simulink model "ES101A_DiagcMgrProxyX"  (R2013b)
settings: Solver=ode45  StartTime=0.0  StopTime=10.0  RelTol=1e-3
values from neighbouring files (symbols this model uses):
  DFTAGICNTR_CNT_U08 = DataDict.Constant    [ES101A_DiagcMgr_DataDict.m]
  DIAGCMGR_NTCINFOSTSTESTFAILD_CNT_U08 = DataDict.Constant    [ES101A_DiagcMgrProxyX_DataDict.m]    (also in ES101A_DiagcMgr_DataDict.m)
  DIAGCMGR_NTCINFOSTSTESTFAILDTHISIGNCYC_CNT_U08 = DataDict.Constant    [ES101A_DiagcMgr_DataDict.m]
  DIAGCMGR_NTCINFOSTSTESTNOTCMPLTHISIGNCYC_CNT_U08 = DataDict.Constant    [ES101A_DiagcMgrProxyX_DataDict.m]    (also in ES101A_DiagcMgr_DataDict.m)
  DiagcMgrFltResp = DataDict.Calibration    [ES101A_DiagcMgrProxyX_DataDict.m]    (also in ES101A_DiagcMgr_DataDict.m)
  DIAGCSTSDFTHWAG_CNT_U16 = DataDict.Constant    [ES101A_DiagcMgr_DataDict.m]
  DIAGCSTSDFTHWAGSERLCOMEXPRTVAL_CNT_U16 = DataDict.Constant    [ES101A_DiagcMgr_DataDict.m]
  DIAGCSTSDFTVEHSPD_CNT_U16 = DataDict.Constant    [ES101A_DiagcMgr_DataDict.m]
  DIAGCSTSININVAL_CNT_U16 = DataDict.Constant    [ES101A_DiagcMgrProxyX_DataDict.m]    (also in ES101A_DiagcMgr_DataDict.m)
  DIAGCSTSIVTR1INACTV_CNT_U16 = DataDict.Constant    [ES101A_DiagcMgr_DataDict.m]
  DIAGCSTSIVTR2INACTV_CNT_U16 = DataDict.Constant    [ES101A_DiagcMgr_DataDict.m]
  DIAGCSTSLIMDTPRFMNC_CNT_U16 = DataDict.Constant    [ES101A_DiagcMgr_DataDict.m]
  DIAGCSTSWHLIMBREJCTNDI_CNT_U16 = DataDict.Constant    [ES101A_DiagcMgr_DataDict.m]
  ELECGLBPRM_IVTRCNT_CNT_U08 = DataDict.ConfigParam    [ES101A_DiagcMgrProxyX_DataDict.m]    (also in ES101A_DiagcMgr_DataDict.m)
  MAXRAMPRATE_ULSPERSEC_F32 = DataDict.Constant    [ES101A_DiagcMgrProxyX_DataDict.m]    (also in ES101A_DiagcMgr_DataDict.m)
  MINRAMPRATE_ULSPERSEC_F32 = DataDict.Constant    [ES101A_DiagcMgrProxyX_DataDict.m]    (also in ES101A_DiagcMgr_DataDict.m)
  SCAMOTTQCMDTOONE_ULS_F32 = DataDict.Constant    [ES101A_DiagcMgrProxyX_DataDict.m]    (also in ES101A_DiagcMgr_DataDict.m)
  SCAMOTTQCMDTOZERO_ULS_F32 = DataDict.Constant    [ES101A_DiagcMgrProxyX_DataDict.m]    (also in ES101A_DiagcMgr_DataDict.m)
undefined symbols (not defined in the file or in its folder): ActvMotTqCmdSca, ActvRampRate, AgiCntr, DIAGCMGR_APPLIDXX_CNT_U08, DiagcMgrNtcMap, DiagcSts, NtcStInfo, Sts
libraries: simulink x21
(part 1 of 3)
settings Model: Creator=nzg49t  LastModifiedBy=nzg49t

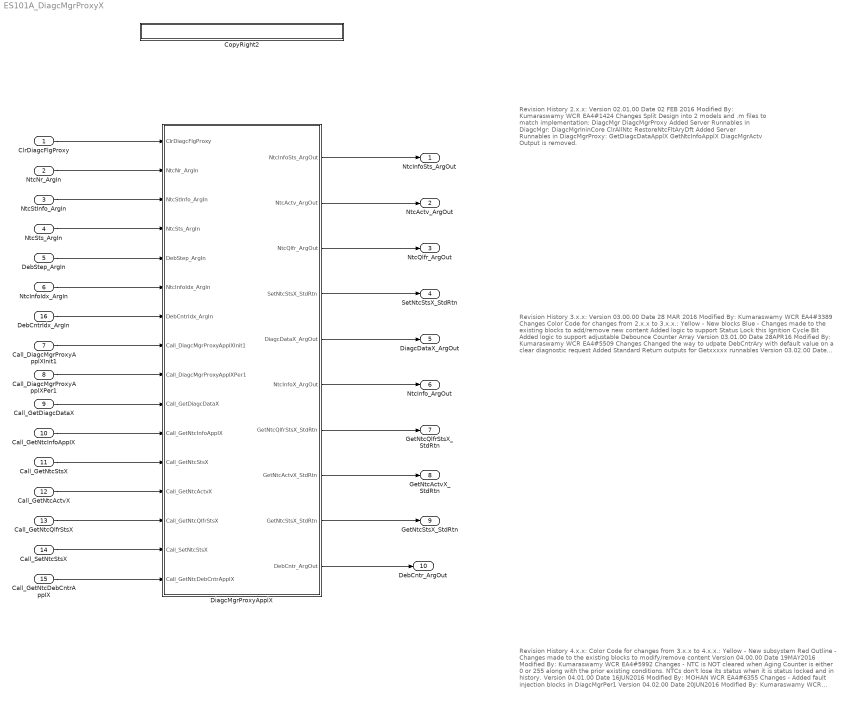
== system ES101A_DiagcMgrProxyX ==
  note: Revision History 2.x.x:
      |
      | Version		02.01.00
      | Date 		02 FEB 2016
      | Modified By: 	Kumaraswamy
      | WCR		EA4#1424
      | Changes		Split Design into 2 models and .m files to match implementation:
      | 				DiagcMgr
      | 				DiagcMgrProxy
      | 			Added Server Runnables in DiagcMgr:
      | 				DiagcMgrIninCore
      | 				ClrAllNtc
      | 				RestoreNtcFltAryDft
      | 			Added Server Runnables in DiagcMgrProxy:
      | 				GetDiagcDataApplX
      | 				GetNtcInfoApplX
      | 			DiagcMgrActv Output is removed.
  note: Revision History 3.x.x:
      |
      | Version		03.00.00
      | Date 		28 MAR 2016
      | Modified By: 	Kumaraswamy
      | WCR		EA4#3389
      | Changes		Color Code for changes from 2.x.x to 3.x.x.:
      | 			Yellow -  New blocks
      | 			Blue -  Changes made to the existing blocks to add/remove new content
      | 			Added logic to support Status Lock this Ignition Cycle Bit
      | 			Added logic to support adjustable Debounce Counter Array
      |
      | Version		03.01.00
      | Date 		28APR16
      | Modified By: 	Kumaraswamy
      | WCR		EA4#5509
      | Changes		Changed the way to udpate DebCntrAry with default value on a clear diagnostic request
      | 			Added Standard Return outputs for Getxxxxx runnables
      |
      | Version		03.02.00
      | Date 		29APR16
      | Modified By: 	Kumaraswamy
      | WCR		EA4#5509
      | Changes		Matched the PrevClrDtcFlg, ClrDtcFlg, ClrDiagcFlgProxy, PrevClrNtcFlgX to have a DataType of Boolean in .m file
      | 			Added GetNtcxxx_StdRtn to all the GetNtcxxx functions
  note: Revision History 4.x.x:
      |
      | Color Code for changes from 3.x.x to 4.x.x.:
      | 	Yellow -  New subsystem
      | 	Red Outline -  Changes made to the existing blocks to modify/remove content
      |
      | Version		04.00.00
      | Date 		19MAY2016
      | Modified By: 	Kumaraswamy
      | WCR		EA4#5992
      | Changes		- NTC is NOT cleared when Aging Counter is either 0 or 255 along with the prior existing conditions.
      | 			NTCs don't lose its status when it is status locked and in history.
      |
      | Version		04.01.00
      | Date 		16JUN2016
      | Modified By: 	MOHAN
      | WCR		EA4#6355
      | Changes		- Added fault injection blocks in DiagcMgrPer1
      |
      | Version		04.02.00
      | Date 		20JUN2016
      | Modified By: 	Kumaraswamy
      | WCR		EA4#6360
      | Changes		- Changed call to the DEM: Clear all DTCs in DiagcMgrPer2
      | 			- Loop counter datatype changed from int32 to int16 in RestoreSnpshtAryDft
      | 			- RestoreSnpshtAryDft and RestoreNtcFltAryDft
      | 			- Added new server Runnable GetNtcDebCntrAppIX to read the Debounce counter of any NTC in application X
      |
      | Version		04.02.01
      | Date 		29JUN2016
      | Modified By: 	Kumaraswamy
      | WCR		EA4#
      | Changes		NO CHANGES TO PROXY. CHANGES TO DIAGCMGRCORE INCLUDES THE FOLLOWING:
      | 			- Removed Data Type Convert blocks when loading 0s to NvM Block of SnpshtAry in RestoreSnpshtAryDft
      | 			- Added output out of the Defalt Case Switch Statement in Per2 for all NTCs
      | 			- Added a condition in If to check if DTC Idx is less than or equal to TOTNROFDTC_CNT_U08 in Per2
      | 			- ClrSnpshtData loaded with correct defualt values
      |
      | Version		04.03.00
      | Date 		15AUG2016
      | Modified By: 	Kumaraswamy
      | WCR		EA4#6904
      | Changes		- PIL Optimizations
      |
      | Version		04.04.00
      | Date 		14SEP2016
      | Modified By: 	Kumaraswamy
      | WCR		EA4#7573
      | Changes		- Overflow condition averted in PreFaild
      | 			- No Changes in Proxy
  ClrDiagcFlgProxy : Inport
  NtcNr_ArgIn : Inport  Port=2
  NtcStInfo_ArgIn : Inport  Port=3
  NtcSts_ArgIn : Inport  Port=4
  DebStep_ArgIn : Inport  Port=5
  NtcInfoIdx_ArgIn : Inport  Port=6
  Call_DiagcMgrProxyApplXInit1 : Inport  Port=7
  Call_DiagcMgrProxyApplXPer1 : Inport  Port=8
  Call_GetDiagcDataX : Inport  Port=9
  Call_GetNtcInfoAppIX : Inport  Port=10
  Call_GetNtcStsX : Inport  Port=11
  Call_GetNtcActvX : Inport  Port=12
  Call_GetNtcQlfrStsX : Inport  Port=13
  Call_SetNtcStsX : Inport  Port=14
  Call_GetNtcDebCntrAppIX : Inport  Port=15
  DebCntrIdx_ArgIn : Inport  Port=16
  CopyRight2 : Subsystem  Description=|  mask(Copyright Information){none=on}
      | Copyright info block.                                               
      |                                                                     
      | Place copyright information at the top of every subsystem in design.
      mask prompts: none "No parameters"
      mask help: Place copyright information at the top of every subsystem in design.
      mask Display:
      | NxtrConf = 'Nexteer Confidential';
      | 
      | sys = bdroot; %handle for the current model ("system")
      | first = get_param(sys,'Created');
      | first = first(end-3:end);  %year is last four digits
      | 
      | last = get_param(sys,'LastModifiedDate');
      | if isempty(last)
      |     last = datestr(now,'yyyy');
      | else
      |     last = last(end-3:end);
      | end
      | 
      | if strcmp(first,last)
      |     fprintf('%s -- Copyright %s Nexteer',NxtrConf,first)
      | else
      |     fprintf('%s -- %s%s- %s Nexteer',NxtrConf,char(169),first,last)
      | end
  DiagcMgrProxyApplX : Subsystem  RequirementInfo="{'linktype_rmi_doors' '0000c474 (/ESG Group/FDD Module Requirements/EA4 Specific/ES101A_DiagcMgr)' '#ES101A_16' 'true' 'REQ:  ES101A_16' '' } %GIDa_0f0e57dd_77ff_4595_8f5a_e90f5f57bb65"
  NtcInfoSts_ArgOut : Outport
  NtcActv_ArgOut : Outport  Port=2
  NtcQlfr_ArgOut : Outport  Port=3
  SetNtcStsX_StdRtn : Outport  Port=4
  DiagcDataX_ArgOut : Outport  Port=5
  NtcInfo_ArgOut : Outport  Port=6
  GetNtcQlfrStsX_StdRtn : Outport  Port=7
  GetNtcActvX_StdRtn : Outport  Port=8
  GetNtcStsX_StdRtn : Outport  Port=9
  DebCntr_ArgOut : Outport  Port=10
  wires:
  NtcNr_ArgIn/1 -> DiagcMgrProxyApplX/2(NtcNr_ArgIn)
  NtcStInfo_ArgIn/1 -> DiagcMgrProxyApplX/3(NtcStInfo_ArgIn)
  NtcSts_ArgIn/1 -> DiagcMgrProxyApplX/4(NtcSts_ArgIn)
  DebStep_ArgIn/1 -> DiagcMgrProxyApplX/5("DebStep_ArgIn ")
  NtcInfoIdx_ArgIn/1 -> DiagcMgrProxyApplX/6(NtcInfoIdx_ArgIn)
  ClrDiagcFlgProxy/1 -> DiagcMgrProxyApplX/1(ClrDiagcFlgProxy)
  DiagcMgrProxyApplX/6(NtcInfoX_ArgOut) -> NtcInfo_ArgOut/1
  DiagcMgrProxyApplX/5(DiagcDataX_ArgOut) -> DiagcDataX_ArgOut/1
  DiagcMgrProxyApplX/4(SetNtcStsX_StdRtn) -> SetNtcStsX_StdRtn/1
  DiagcMgrProxyApplX/1(NtcInfoSts_ArgOut) -> NtcInfoSts_ArgOut/1
  DiagcMgrProxyApplX/2(NtcActv_ArgOut) -> NtcActv_ArgOut/1
  DiagcMgrProxyApplX/3(NtcQlfr_ArgOut) -> NtcQlfr_ArgOut/1
  Call_DiagcMgrProxyApplXInit1/1 -> DiagcMgrProxyApplX/8(Call_DiagcMgrProxyApplXInit1)
  Call_DiagcMgrProxyApplXPer1/1 -> DiagcMgrProxyApplX/9(Call_DiagcMgrProxyApplXPer1)
  Call_GetDiagcDataX/1 -> DiagcMgrProxyApplX/10(Call_GetDiagcDataX)
  Call_GetNtcInfoAppIX/1 -> DiagcMgrProxyApplX/11(Call_GetNtcInfoAppIX)
  Call_GetNtcStsX/1 -> DiagcMgrProxyApplX/12(Call_GetNtcStsX)
  Call_GetNtcActvX/1 -> DiagcMgrProxyApplX/13(Call_GetNtcActvX)
  Call_GetNtcQlfrStsX/1 -> DiagcMgrProxyApplX/14(Call_GetNtcQlfrStsX)
  Call_SetNtcStsX/1 -> DiagcMgrProxyApplX/15(Call_SetNtcStsX)
  DiagcMgrProxyApplX/9(GetNtcStsX_StdRtn) -> GetNtcStsX_StdRtn/1
  DiagcMgrProxyApplX/8(GetNtcActvX_StdRtn) -> GetNtcActvX_StdRtn/1
  DiagcMgrProxyApplX/7(GetNtcQlfrStsX_StdRtn) -> GetNtcQlfrStsX_StdRtn/1
  Call_GetNtcDebCntrAppIX/1 -> DiagcMgrProxyApplX/16(Call_GetNtcDebCntrAppIX)
  DebCntrIdx_ArgIn/1 -> DiagcMgrProxyApplX/7(DebCntrIdx_ArgIn)
  DiagcMgrProxyApplX/10(DebCntr_ArgOut) -> DebCntr_ArgOut/1

== system ES101A_DiagcMgrProxyX/CopyRight2 ==

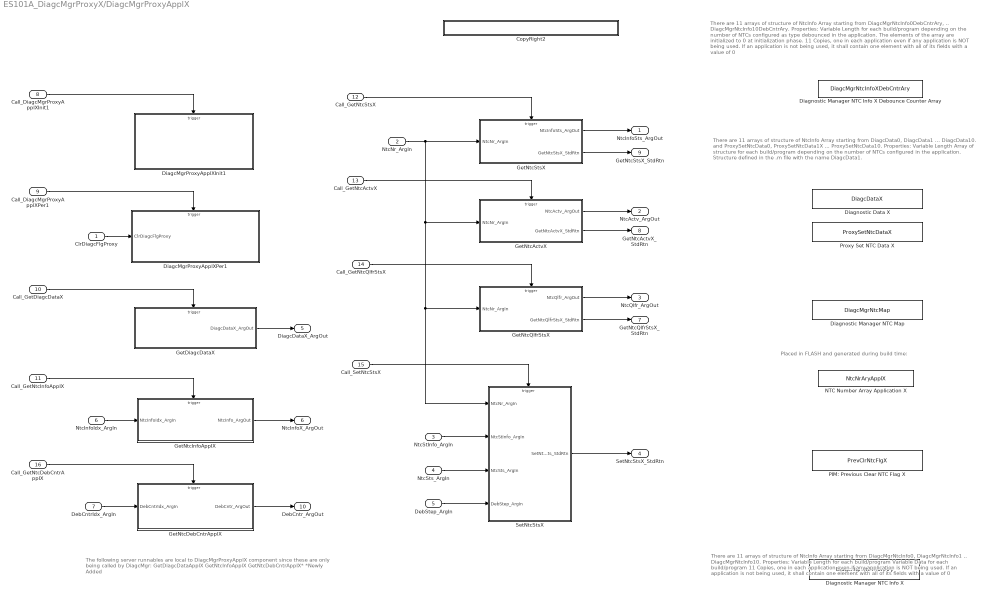
== system ES101A_DiagcMgrProxyX/DiagcMgrProxyApplX ==
  note: There are 11 arrays of structure of NtcInfo Array starting from DiagcMgrNtcInfo0DebCntrAry, .. DiagcMgrNtcInfo10DebCntrAry.
      | 	Properties:
      | 		Variable Length for each build/program depending on the number of NTCs configured as type debounced in the application.
      | 		The elements of the array are initialized to 0 at initialization phase.
      | 		11 Copies, one in each application even if any application is NOT being used.
      | 		If an application is not being used, it shall contain one element with all of its fields with a value of 0
  note: Placed in FLASH and generated during build time:
  note: There are 11 arrays of structure of NtcInfo Array starting from DiagcMgrNtcInfo0, DiagcMgrNtcInfo1 .. DiagcMgrNtcInfo10.
      | 	Properties:
      | 		Variable Length for each build/program
      | 		Variable Data for each build/program
      | 		11 Copies, one in each application even if any application is NOT being used.
      | 		If an application is not being used, it shall contain one element with all of its fields with a value of 0
  note: There are 11 arrays of structure of NtcInfo Array starting from DiagcData0, DiagcData1 ... DiagcData10.
      | 	and 	ProxySetNtcData0, ProxySetNtcData1X ... ProxySetNtcData10.
      | 	Properties:
      | 		Variable Length Array of structure for each build/program depending on the number of NTCs configured in the application.
      | 		Structure defined in the .m file with the name DiagcData1.
  note: The following server runnables are local to DiagcMgrProxyApplX component since these are
      | only being called by DiagcMgr:
      |
      | 	GetDiagcDataApplX
      | 	GetNtcInfoApplX
      | 	GetNtcDebCntrAppIX*
      |
      | *Newly Added
  ClrDiagcFlgProxy : Inport
  NtcNr_ArgIn : Inport  Port=2
  NtcStInfo_ArgIn : Inport  Port=3
  NtcSts_ArgIn : Inport  Port=4
  "DebStep_ArgIn " : Inport  Port=5
  NtcInfoIdx_ArgIn : Inport  Port=6
  DebCntrIdx_ArgIn : Inport  Port=7
  Call_DiagcMgrProxyApplXInit1 : Inport  Port=8
  Call_DiagcMgrProxyApplXPer1 : Inport  Port=9
  Call_GetDiagcDataX : Inport  Port=10
  Call_GetNtcInfoAppIX : Inport  Port=11
  Call_GetNtcStsX : Inport  Port=12
  Call_GetNtcActvX : Inport  Port=13
  Call_GetNtcQlfrStsX : Inport  Port=14
  Call_SetNtcStsX : Inport  Port=15
  Call_GetNtcDebCntrAppIX : Inport  Port=16
  CopyRight2 : Subsystem  Description=|  mask(Copyright Information){none=on}
      | Copyright info block.                                               
      |                                                                     
      | Place copyright information at the top of every subsystem in design.
      mask prompts: none "No parameters"
      mask help: Place copyright information at the top of every subsystem in design.
      mask Display:
      | NxtrConf = 'Nexteer Confidential';
      | 
      | sys = bdroot; %handle for the current model ("system")
      | first = get_param(sys,'Created');
      | first = first(end-3:end);  %year is last four digits
      | 
      | last = get_param(sys,'LastModifiedDate');
      | if isempty(last)
      |     last = datestr(now,'yyyy');
      | else
      |     last = last(end-3:end);
      | end
      | 
      | if strcmp(first,last)
      |     fprintf('%s -- Copyright %s Nexteer',NxtrConf,first)
      | else
      |     fprintf('%s -- %s%s- %s Nexteer',NxtrConf,char(169),first,last)
      | end
  DiagcMgrProxyApplXInit1 : Subsystem  TreatAsAtomicUnit=on
  DiagcMgrProxyApplXPer1 : Subsystem  Description=|  RequirementInfo={} %GIDa_a74dc586_0f2f_4605_81c6_bcaeb03901b9
      | 10ms
      | Build DiagcSts
      settings: AttributesFormatString=%<Description>
  Diagnostic Data X : DataStoreMemory  DataStoreName=DiagcDataX  InitialValue=[0]  OutDataTypeStr=Bus: DiagcData1  StateMustResolveToSignalObject=on
  Diagnostic Manager NTC Info X : DataStoreMemory  Description=|  RequirementInfo={} %GIDa_1a7b9fd6_aed8_468a_989b_0e93f4940b59  DataStoreName=DiagcMgrNtcInfoXAry  InitialValue=[0 0 0 0 0 0 0 0 0 0 0 0 0 0]  OutDataTypeStr=Bus: NtcInfoRec4  StateMustResolveToSignalObject=on
      | Length is a ConfigParam in ApplNtcCnt.
      | ApplNtcCnt is a table, each index contains 
      | number of NTC for that application.
      settings: AttributesFormatString=%<Description>
  Diagnostic Manager NTC Info X Debounce Counter Array : DataStoreMemory  DataStoreName=DiagcMgrNtcInfoXDebCntrAry  ReadBeforeWriteMsg=warning  WriteAfterWriteMsg=warning  WriteAfterReadMsg=warning  InitialValue=[0 0 0 0 0 0 0 0 0 0 0 0 0 0 0 0]  OutDataTypeStr=int16  StateMustResolveToSignalObject=on
      settings: AttributesFormatString=%<Description>
  Diagnostic Manager NTC Map : DataStoreMemory  Description=|  RequirementInfo={} %GIDa_04e5e147_8331_48b3_8385_fcc35421587e  DataStoreName=DiagcMgrNtcMap  InitialValue=[0 0 0 0 0 0 0 0 0 0 0 0 0 0 0 0 0 0 0 0 0 0 0 0 0 0 0 0 0 0 0 0 0 0 0 0 0 0 0 0 0 0 0 0 0 0 0 0 0 0 0 0 0 0 0 0 0 0 0 0 0 0 0 0 0 0 0 0 0 0 0 0 0 0 0 0 0 0 0 0 0 0 0 0 0 0 0 0 0 0 0 0 0 0 0 0 0 0 0 0 0 0 0 0 0 0 0 0 0 0 0 0 0 0 0 0 0 0 0 0 0 0 0 0 0 0 0 0 0 0 0 0 0 0 0 0 0 0 0 0 0 0 0 0 0 0 0 0 0 0 0 0 0 0 0 0 0 0 0 0 0 0 0 0 0 0 0 0 0 0 0 0 0 0 0 0 0 0 0 0 0 0 0 0 0 0 0 0 0 0 0 0 0 0 0 0 0 0 0 0 0 0 0 0 0 0 0 0 0 0 0 0 0 0 0 0 0 0 0 0 0 0 0 0 0 0 0 0 0 0 0 0 0 0 0 0 0 0 0 0 0 0 0 0 0 0 0 0 0 0 0 0 0 0 0 0 0 0 0 0 0 0 0 0 0 0 0 0 0 0 0 0 0 0 0 0 0 0 0 0 0 0 0 0 0 0 0 0 0 0 0 0 0 0 0 0 0 0 0 0 0 0 0 0 0 0 0 0 0 0 0 0 0 0 0 0 0 0 0 0 0 0 0 0 0 0 0 0 0 0 0 0 0 0 0 0 0 0 0 0 0 0 0 0 0 0 0 0 0 0 0 0 0 0 0 0 0 0 0 0 0 0 0 0 0 0 0 0 0 0 0 0 0 0 0 0 0 0 0 0 0 0 0 0 0 0 0 0 0 0 0 0 0 0 0 0 0 0 0 0 0 0 0 0 0 0 0 0 0 0 0 0 0 0 0 0 0 0 0 0 0 0 0 0 0 0 0 0 0 0 0 0 0 0 0 0 0 0 0 0 0 0 0 0 0 0 0 0 0 0 0 0 0 0 0 0 0 0 0 0 0 0 0 0 0 0 0 0 0 0 0 0 0 0 0 0 0 0 0 0 0 0 0 0 0 0 0 0 0 0 0 0 0 0 0 0 0 0 0 0 0 0 0 0 0 0 0 0 0 0 0 0]  OutDataTypeStr=Bus: NtcMapRec2
      | FOR SIMULATION ONLY! 
      | Will be generated during build time.
      | Configurable Constant
      | Constant Length
      | Variable Data
      settings: AttributesFormatString=%<Description>
  "GetDiagcDataX " : Subsystem  Description=Can only be called from 2ms Periodics since it doesn't use an EXCLUSIVE AREA.  RequirementInfo={} %GIDa_576594b7_7567_4d5f_b9cd_6ed2a69f402f
      settings: AttributesFormatString=%<Description>
  GetNtcActvX : Subsystem  RequirementInfo="{'linktype_rmi_doors' '0000c474 (/ESG Group/FDD Module Requirements/EA4 Specific/ES101A_DiagcMgr)' '#ES101A_144' 'true' 'REQ:  ES101A_144' '' } %GIDa_6f53a8ff_e049_484a_8f6f_85fe6fb9e2f0"  TreatAsAtomicUnit=on
      settings: AttributesFormatString=%<Description>
  GetNtcDebCntrApplX : Subsystem  TreatAsAtomicUnit=on
  GetNtcInfoAppIX : Subsystem  TreatAsAtomicUnit=on
  GetNtcQlfrStsX : Subsystem  RequirementInfo="{'linktype_rmi_doors' '0000c474 (/ESG Group/FDD Module Requirements/EA4 Specific/ES101A_DiagcMgr)' '#ES101A_74' 'true' 'REQ:  ES101A_74' '' } %GIDa_4890291f_9b5c_4c6f_ba8d_b8498b56473b"  TreatAsAtomicUnit=on
      settings: AttributesFormatString=%<Description>
  GetNtcStsX : Subsystem  RequirementInfo="{'linktype_rmi_doors' '0000c474 (/ESG Group/FDD Module Requirements/EA4 Specific/ES101A_DiagcMgr)' '#ES101A_72' 'true' 'REQ:  ES101A_72' '' } %GIDa_d58b09bb_926c_4698_b92b_8f64a4f0a7f3"  TreatAsAtomicUnit=on
      settings: AttributesFormatString=%<Description>
  NTC Number Array Application X : DataStoreMemory  Description=|  DataStoreName=NtcNrAryApplX  ReadBeforeWriteMsg=warning  WriteAfterWriteMsg=warning  WriteAfterReadMsg=warning  InitialValue=[1 2 3 4 5 6 7 8 9 10 11 12 13 14]  OutDataTypeStr=uint16
      | Size is based on the number of the NTCs present in the Application.
      | It contains the list of NTCs in each application.
      settings: AttributesFormatString=%<Description>
  PIM: Previous Clear NTC Flag X : DataStoreMemory  DataStoreName=PrevClrNtcFlgX  InitialValue=[0]  OutDataTypeStr=uint8  StateMustResolveToSignalObject=on
  Proxy Set NTC Data X : DataStoreMemory  DataStoreName=ProxySetNtcDataX  InitialValue=[0]  OutDataTypeStr=Bus: DiagcData1  StateMustResolveToSignalObject=on
  SetNtcStsX : Subsystem  TreatAsAtomicUnit=on
  NtcInfoSts_ArgOut : Outport
  NtcActv_ArgOut : Outport  Port=2
  NtcQlfr_ArgOut : Outport  Port=3
  SetNtcStsX_StdRtn : Outport  Port=4
  DiagcDataX_ArgOut : Outport  Port=5
  NtcInfoX_ArgOut : Outport  Port=6
  GetNtcQlfrStsX_StdRtn : Outport  Port=7
  GetNtcActvX_StdRtn : Outport  Port=8
  GetNtcStsX_StdRtn : Outport  Port=9
  DebCntr_ArgOut : Outport  Port=10
  wires:
  ClrDiagcFlgProxy/1 -> DiagcMgrProxyApplXPer1/1(ClrDiagcFlgProxy)
  Call_DiagcMgrProxyApplXPer1/1 -> DiagcMgrProxyApplXPer1/Trigger
  Call_DiagcMgrProxyApplXInit1/1 -> DiagcMgrProxyApplXInit1/Trigger
  GetNtcStsX/1(NtcInfoSts_ArgOut) -> NtcInfoSts_ArgOut/1
  GetNtcActvX/1(NtcActv_ArgOut) -> NtcActv_ArgOut/1
  GetNtcQlfrStsX/1(NtcQlfr_ArgOut) -> NtcQlfr_ArgOut/1
  SetNtcStsX/1(SetNtcSts_StdRtn) -> SetNtcStsX_StdRtn/1
  NtcStInfo_ArgIn/1 -> SetNtcStsX/2(NtcStInfo_ArgIn)
  NtcSts_ArgIn/1 -> SetNtcStsX/3(NtcSts_ArgIn)
  "DebStep_ArgIn "/1 -> SetNtcStsX/4(DebStep_ArgIn)
  "GetDiagcDataX "/1(DiagcDataX_ArgOut) -> DiagcDataX_ArgOut/1
  NtcInfoIdx_ArgIn/1 -> GetNtcInfoAppIX/1(NtcInfoIdx_ArgIn)
  GetNtcInfoAppIX/1(NtcInfo_ArgOut) -> NtcInfoX_ArgOut/1
  Call_GetDiagcDataX/1 -> "GetDiagcDataX "/Trigger
  Call_GetNtcInfoAppIX/1 -> GetNtcInfoAppIX/Trigger
  Call_GetNtcStsX/1 -> GetNtcStsX/Trigger
  Call_GetNtcActvX/1 -> GetNtcActvX/Trigger
  Call_GetNtcQlfrStsX/1 -> GetNtcQlfrStsX/Trigger
  Call_SetNtcStsX/1 -> SetNtcStsX/Trigger
  GetNtcStsX/2(GetNtcStsX_StdRtn) -> GetNtcStsX_StdRtn/1
  GetNtcActvX/2(GetNtcActvX_StdRtn) -> GetNtcActvX_StdRtn/1
  GetNtcQlfrStsX/2(GetNtcQlfrStsX_StdRtn) -> GetNtcQlfrStsX_StdRtn/1
  NtcNr_ArgIn/1 -> SetNtcStsX/1(NtcNr_ArgIn), GetNtcQlfrStsX/1(NtcNr_ArgIn), GetNtcActvX/1(NtcNr_ArgIn), GetNtcStsX/1(NtcNr_ArgIn)
  Call_GetNtcDebCntrAppIX/1 -> GetNtcDebCntrApplX/Trigger
  DebCntrIdx_ArgIn/1 -> GetNtcDebCntrApplX/1(DebCntrIdx_ArgIn)
  GetNtcDebCntrApplX/1(DebCntr_ArgOut) -> DebCntr_ArgOut/1

== system ES101A_DiagcMgrProxyX/DiagcMgrProxyApplX/CopyRight2 ==

== system ES101A_DiagcMgrProxyX/DiagcMgrProxyApplX/DiagcMgrProxyApplXInit1 ==
  Function : TriggerPort  TriggerType=function-call  OutputDataType=double
  ApplIdx : Constant  Value=DIAGCMGR_APPLIDXX_CNT_U08
  CopyRight2 : Subsystem  Description=|  mask(Copyright Information){none=on}
      | Copyright info block.                                               
      |                                                                     
      | Place copyright information at the top of every subsystem in design.
      mask prompts: none "No parameters"
      mask help: Place copyright information at the top of every subsystem in design.
      mask Display:
      | NxtrConf = 'Nexteer Confidential';
      | 
      | sys = bdroot; %handle for the current model ("system")
      | first = get_param(sys,'Created');
      | first = first(end-3:end);  %year is last four digits
      | 
      | last = get_param(sys,'LastModifiedDate');
      | if isempty(last)
      |     last = datestr(now,'yyyy');
      | else
      |     last = last(end-3:end);
      | end
      | 
      | if strcmp(first,last)
      |     fprintf('%s -- Copyright %s Nexteer',NxtrConf,first)
      | else
      |     fprintf('%s -- %s%s- %s Nexteer',NxtrConf,char(169),first,last)
      | end
  Data Store Read1 : DataStoreRead  DataStoreName=DiagcMgrNtcInfoXAry
  Data Store Write : DataStoreWrite  DataStoreName=ProxySetNtcDataX
  Data Store Write1 : DataStoreWrite  DataStoreName=DiagcDataX
  Data Store Write2 : DataStoreWrite  DataStoreName=DiagcMgrNtcInfoXAry
  DiagcMgrIninCore : Subsystem
  Width : Width  DataType=uint8
  wires:
  Width/1 -> DiagcMgrIninCore/2(NtcInfoArySize_ArgIn)
  ApplIdx/1 -> DiagcMgrIninCore/1(AppIdx_ArgIn)
  DiagcMgrIninCore/1(DiagcData_ArgOut) -> Data Store Write1/1
  DiagcMgrIninCore/2(ProxySetNtcData_ArgOut) -> Data Store Write/1
  DiagcMgrIninCore/3(NtcInfoAry_ArgOut) -> Data Store Write2/1
  Data Store Read1/1 -> DiagcMgrIninCore/3(NtcInfoAry_ArgIn), Width/1

== system ES101A_DiagcMgrProxyX/DiagcMgrProxyApplX/DiagcMgrProxyApplXPer1 ==
  note: DiagcMgr model is using the following DataStore units as a temporary variables. These will not be shown in the .m file since they're not PIM, but they shall be coded as these are used in the Per1.
      | This method is used to save some memory for the static variables.
  ClrDiagcFlgProxy : Inport
  Function : TriggerPort  TriggerType=function-call  OutputDataType=double
  Clear All NTCs : Subsystem  TreatAsAtomicUnit=on
  CopyRight2 : Subsystem  Description=|  mask(Copyright Information){none=on}
      | Copyright info block.                                               
      |                                                                     
      | Place copyright information at the top of every subsystem in design.
      mask prompts: none "No parameters"
      mask help: Place copyright information at the top of every subsystem in design.
      mask Display:
      | NxtrConf = 'Nexteer Confidential';
      | 
      | sys = bdroot; %handle for the current model ("system")
      | first = get_param(sys,'Created');
      | first = first(end-3:end);  %year is last four digits
      | 
      | last = get_param(sys,'LastModifiedDate');
      | if isempty(last)
      |     last = datestr(now,'yyyy');
      | else
      |     last = last(end-3:end);
      | end
      | 
      | if strcmp(first,last)
      |     fprintf('%s -- Copyright %s Nexteer',NxtrConf,first)
      | else
      |     fprintf('%s -- %s%s- %s Nexteer',NxtrConf,char(169),first,last)
      | end
  Data Store Memory1 : DataStoreMemory  DataStoreName=ProxyPerData  InitialValue=[0]  OutDataTypeStr=Bus: DiagcData1
  Data Store Read : DataStoreRead  DataStoreName=PrevClrNtcFlgX
  Data Store Read1 : DataStoreRead  DataStoreName=DiagcMgrNtcInfoXAry
  If : If  NumInputs=2  IfExpression=u1 ~= u2
  Update the DiagcSts : Subsystem  RequirementInfo="{'linktype_rmi_doors' '0000c474 (/ESG Group/FDD Module Requirements/EA4 Specific/ES101A_DiagcMgr)' '#ES101A_208' 'true' 'REQ:  ES101A_208' '' ; 'linktype_rmi_doors' '0000c474 (/ESG Group/FDD Module Requirements/EA4 Specific/ES101A_DiagcMgr)' '#ES101A_209' 'true' 'REQ:  ES101A_209' '' } %GIDa_fac1e9a2_6502_4ec9_9318_60e54df68400"  TreatAsAtomicUnit=on
  Width : Width  DataType=uint8
  wires:
  ClrDiagcFlgProxy/1 -> Clear All NTCs/1(ClrNtcFlg), If/1
  Data Store Read/1 -> If/2
  If/1 -> Clear All NTCs/Action
  If/2 -> Update the DiagcSts/Action
  Data Store Read1/1 -> Width/1
  Width/1 -> Clear All NTCs/2(Number of Iterations), Update the DiagcSts/1(Number of Iterations)

== system ES101A_DiagcMgrProxyX/DiagcMgrProxyApplX/GetDiagcDataX  ==
  Function : TriggerPort  TriggerType=function-call  OutputDataType=double
  CopyRight2 : Subsystem  Description=|  mask(Copyright Information){none=on}
      | Copyright info block.                                               
      |                                                                     
      | Place copyright information at the top of every subsystem in design.
      mask prompts: none "No parameters"
      mask help: Place copyright information at the top of every subsystem in design.
      mask Display:
      | NxtrConf = 'Nexteer Confidential';
      | 
      | sys = bdroot; %handle for the current model ("system")
      | first = get_param(sys,'Created');
      | first = first(end-3:end);  %year is last four digits
      | 
      | last = get_param(sys,'LastModifiedDate');
      | if isempty(last)
      |     last = datestr(now,'yyyy');
      | else
      |     last = last(end-3:end);
      | end
      | 
      | if strcmp(first,last)
      |     fprintf('%s -- Copyright %s Nexteer',NxtrConf,first)
      | else
      |     fprintf('%s -- %s%s- %s Nexteer',NxtrConf,char(169),first,last)
      | end
  Data Store Read : DataStoreRead  DataStoreName=DiagcDataX
  DiagcDataX_ArgOut : Outport
  wires:
  Data Store Read/1 -> DiagcDataX_ArgOut/1

== system ES101A_DiagcMgrProxyX/DiagcMgrProxyApplX/GetNtcActvX ==
  NtcNr_ArgIn : Inport
  Function : TriggerPort  TriggerType=function-call  OutputDataType=double
  CopyRight2 : Subsystem  Description=|  mask(Copyright Information){none=on}
      | Copyright info block.                                               
      |                                                                     
      | Place copyright information at the top of every subsystem in design.
      mask prompts: none "No parameters"
      mask help: Place copyright information at the top of every subsystem in design.
      mask Display:
      | NxtrConf = 'Nexteer Confidential';
      | 
      | sys = bdroot; %handle for the current model ("system")
      | first = get_param(sys,'Created');
      | first = first(end-3:end);  %year is last four digits
      | 
      | last = get_param(sys,'LastModifiedDate');
      | if isempty(last)
      |     last = datestr(now,'yyyy');
      | else
      |     last = last(end-3:end);
      | end
      | 
      | if strcmp(first,last)
      |     fprintf('%s -- Copyright %s Nexteer',NxtrConf,first)
      | else
      |     fprintf('%s -- %s%s- %s Nexteer',NxtrConf,char(169),first,last)
      | end
  Data Store Read : DataStoreRead  DataStoreName=DiagcMgrNtcInfoXAry
  E_OK : Constant  Value=0
  GetNtcActvCore : Subsystem  RequirementInfo={} %GIDa_12e891d0_edf8_4895_8187_662619b71e53
      settings: AttributesFormatString=%<Description>
  NtcActv_ArgOut : Outport
  GetNtcActvX_StdRtn : Outport  Port=2
  wires:
  NtcNr_ArgIn/1 -> GetNtcActvCore/1(NtcNr_ArgIn)
  Data Store Read/1 -> GetNtcActvCore/2(NtcInfoAry_ArgIn)
  GetNtcActvCore/1(NtcActv_ArgOut) -> NtcActv_ArgOut/1
  E_OK/1 -> GetNtcActvX_StdRtn/1

== system ES101A_DiagcMgrProxyX/DiagcMgrProxyApplX/GetNtcDebCntrApplX ==
  DebCntrIdx_ArgIn : Inport
  Function : TriggerPort  TriggerType=function-call  OutputDataType=double
  CopyRight2 : Subsystem  Description=|  mask(Copyright Information){none=on}
      | Copyright info block.                                               
      |                                                                     
      | Place copyright information at the top of every subsystem in design.
      mask prompts: none "No parameters"
      mask help: Place copyright information at the top of every subsystem in design.
      mask Display:
      | NxtrConf = 'Nexteer Confidential';
      | 
      | sys = bdroot; %handle for the current model ("system")
      | first = get_param(sys,'Created');
      | first = first(end-3:end);  %year is last four digits
      | 
      | last = get_param(sys,'LastModifiedDate');
      | if isempty(last)
      |     last = datestr(now,'yyyy');
      | else
      |     last = last(end-3:end);
      | end
      | 
      | if strcmp(first,last)
      |     fprintf('%s -- Copyright %s Nexteer',NxtrConf,first)
      | else
      |     fprintf('%s -- %s%s- %s Nexteer',NxtrConf,char(169),first,last)
      | end
  Data Store Read4 : DataStoreRead  DataStoreName=DiagcMgrNtcInfoXDebCntrAry
  Selector : Selector  IndexMode=Zero-based  InputPortWidth=14  IndexOptions=Index vector (port)  Indices=[1 3]  OutputSizes=1
  DebCntr_ArgOut : Outport
  wires:
  Data Store Read4/1 -> Selector/1
  DebCntrIdx_ArgIn/1 -> Selector/2
  Selector/1 -> DebCntr_ArgOut/1

== system ES101A_DiagcMgrProxyX/DiagcMgrProxyApplX/GetNtcInfoAppIX ==
  NtcInfoIdx_ArgIn : Inport
  Function : TriggerPort  TriggerType=function-call  OutputDataType=double
  CopyRight2 : Subsystem  Description=|  mask(Copyright Information){none=on}
      | Copyright info block.                                               
      |                                                                     
      | Place copyright information at the top of every subsystem in design.
      mask prompts: none "No parameters"
      mask help: Place copyright information at the top of every subsystem in design.
      mask Display:
      | NxtrConf = 'Nexteer Confidential';
      | 
      | sys = bdroot; %handle for the current model ("system")
      | first = get_param(sys,'Created');
      | first = first(end-3:end);  %year is last four digits
      | 
      | last = get_param(sys,'LastModifiedDate');
      | if isempty(last)
      |     last = datestr(now,'yyyy');
      | else
      |     last = last(end-3:end);
      | end
      | 
      | if strcmp(first,last)
      |     fprintf('%s -- Copyright %s Nexteer',NxtrConf,first)
      | else
      |     fprintf('%s -- %s%s- %s Nexteer',NxtrConf,char(169),first,last)
      | end
  Data Store Read : DataStoreRead  DataStoreName=DiagcMgrNtcInfoXAry
  Selector : Selector  IndexMode=Zero-based  InputPortWidth=14  IndexOptions=Index vector (port)  Indices=[1 3]  OutputSizes=1
  NtcInfo_ArgOut : Outport
  wires:
  Data Store Read/1 -> Selector/1
  NtcInfoIdx_ArgIn/1 -> Selector/2
  Selector/1 -> NtcInfo_ArgOut/1

== system ES101A_DiagcMgrProxyX/DiagcMgrProxyApplX/GetNtcQlfrStsX ==
  NtcNr_ArgIn : Inport
  Function : TriggerPort  TriggerType=function-call  OutputDataType=double
  CopyRight2 : Subsystem  Description=|  mask(Copyright Information){none=on}
      | Copyright info block.                                               
      |                                                                     
      | Place copyright information at the top of every subsystem in design.
      mask prompts: none "No parameters"
      mask help: Place copyright information at the top of every subsystem in design.
      mask Display:
      | NxtrConf = 'Nexteer Confidential';
      | 
      | sys = bdroot; %handle for the current model ("system")
      | first = get_param(sys,'Created');
      | first = first(end-3:end);  %year is last four digits
      | 
      | last = get_param(sys,'LastModifiedDate');
      | if isempty(last)
      |     last = datestr(now,'yyyy');
      | else
      |     last = last(end-3:end);
      | end
      | 
      | if strcmp(first,last)
      |     fprintf('%s -- Copyright %s Nexteer',NxtrConf,first)
      | else
      |     fprintf('%s -- %s%s- %s Nexteer',NxtrConf,char(169),first,last)
      | end
  Data Store Read : DataStoreRead  DataStoreName=DiagcMgrNtcInfoXAry
  E_OK : Constant  Value=0
  GetNtcQlfrStsCore : Subsystem  RequirementInfo={} %GIDa_8edbae63_f18c_4e32_a4c5_51d57f6a1bb7
      settings: AttributesFormatString=%<Description>
  NtcQlfr_ArgOut : Outport
  GetNtcQlfrStsX_StdRtn : Outport  Port=2
  wires:
  GetNtcQlfrStsCore/1(NtcQlfr_ArgOut) -> NtcQlfr_ArgOut/1
  Data Store Read/1 -> GetNtcQlfrStsCore/2(NtcInfoAry_ArgIn)
  NtcNr_ArgIn/1 -> GetNtcQlfrStsCore/1(NtcNr_ArgIn)
  E_OK/1 -> GetNtcQlfrStsX_StdRtn/1

== system ES101A_DiagcMgrProxyX/DiagcMgrProxyApplX/GetNtcStsX ==
  NtcNr_ArgIn : Inport
  Function : TriggerPort  TriggerType=function-call  OutputDataType=double
  CopyRight2 : Subsystem  Description=|  mask(Copyright Information){none=on}
      | Copyright info block.                                               
      |                                                                     
      | Place copyright information at the top of every subsystem in design.
      mask prompts: none "No parameters"
      mask help: Place copyright information at the top of every subsystem in design.
      mask Display:
      | NxtrConf = 'Nexteer Confidential';
      | 
      | sys = bdroot; %handle for the current model ("system")
      | first = get_param(sys,'Created');
      | first = first(end-3:end);  %year is last four digits
      | 
      | last = get_param(sys,'LastModifiedDate');
      | if isempty(last)
      |     last = datestr(now,'yyyy');
      | else
      |     last = last(end-3:end);
      | end
      | 
      | if strcmp(first,last)
      |     fprintf('%s -- Copyright %s Nexteer',NxtrConf,first)
      | else
      |     fprintf('%s -- %s%s- %s Nexteer',NxtrConf,char(169),first,last)
      | end
  Data Store Read : DataStoreRead  DataStoreName=DiagcMgrNtcInfoXAry
  E_OK : Constant  Value=0
  GetNtcStsCore : Subsystem  RequirementInfo={} %GIDa_40dac964_d246_44ba_aed1_2f4640d99331
      settings: AttributesFormatString=%<Description>
  NtcInfoSts_ArgOut : Outport
  GetNtcStsX_StdRtn : Outport  Port=2
  wires:
  NtcNr_ArgIn/1 -> GetNtcStsCore/1(NtcNr_ArgIn)
  Data Store Read/1 -> GetNtcStsCore/2(NtcInfoAry_ArgIn)
  GetNtcStsCore/1(NtcInfoSts_ArgOut) -> NtcInfoSts_ArgOut/1
  E_OK/1 -> GetNtcStsX_StdRtn/1

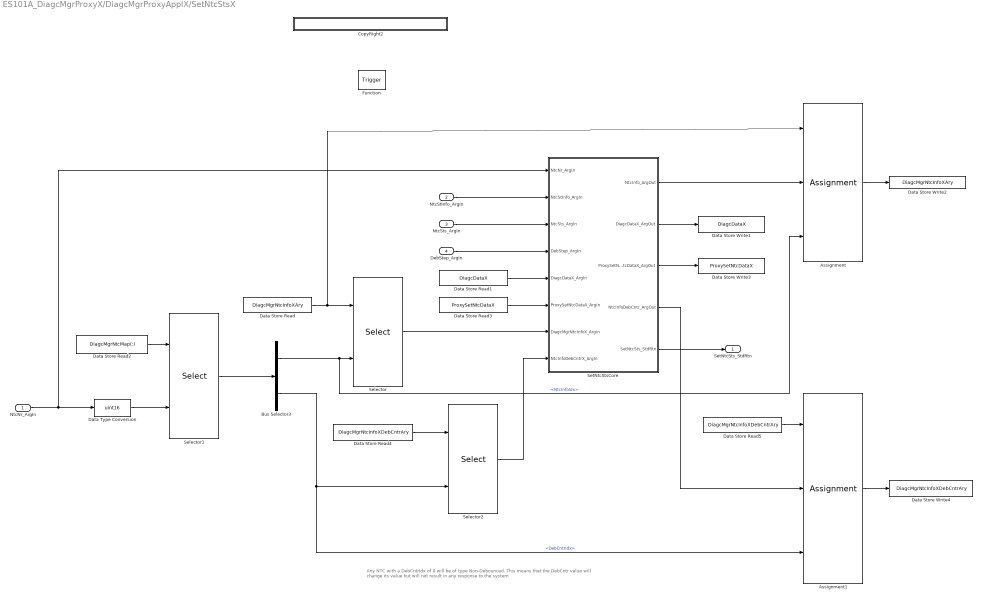
== system ES101A_DiagcMgrProxyX/DiagcMgrProxyApplX/SetNtcStsX ==
  note: Any NTC with a DebCntrIdx of 0 will be of type Non-Debounced.
      | This means that the DebCntr value will change its value but will not result in any response to the system
  NtcNr_ArgIn : Inport
  NtcStInfo_ArgIn : Inport  Port=2
  NtcSts_ArgIn : Inport  Port=3
  DebStep_ArgIn : Inport  Port=4
  Function : TriggerPort  TriggerType=function-call  OutputDataType=double
  Assignment : Assignment  IndexMode=Zero-based  IndexOptions=Index vector (port)  Indices=1  OutputSizes=1
  Assignment1 : Assignment  IndexMode=Zero-based  IndexOptions=Index vector (port)  Indices=1  OutputSizes=1
  Bus Selector3 : BusSelector  OutputSignals=NtcInfoIdx,DebCntrIdx
  CopyRight2 : Subsystem  Description=|  mask(Copyright Information){none=on}
      | Copyright info block.                                               
      |                                                                     
      | Place copyright information at the top of every subsystem in design.
      mask prompts: none "No parameters"
      mask help: Place copyright information at the top of every subsystem in design.
      mask Display:
      | NxtrConf = 'Nexteer Confidential';
      | 
      | sys = bdroot; %handle for the current model ("system")
      | first = get_param(sys,'Created');
      | first = first(end-3:end);  %year is last four digits
      | 
      | last = get_param(sys,'LastModifiedDate');
      | if isempty(last)
      |     last = datestr(now,'yyyy');
      | else
      |     last = last(end-3:end);
      | end
      | 
      | if strcmp(first,last)
      |     fprintf('%s -- Copyright %s Nexteer',NxtrConf,first)
      | else
      |     fprintf('%s -- %s%s- %s Nexteer',NxtrConf,char(169),first,last)
      | end
  Data Store Read : DataStoreRead  DataStoreName=DiagcMgrNtcInfoXAry
  Data Store Read1 : DataStoreRead  DataStoreName=DiagcDataX
  Data Store Read2 : DataStoreRead  DataStoreName=DiagcMgrNtcMap  DataStoreElements=DiagcMgrNtcMap(:)
  Data Store Read3 : DataStoreRead  DataStoreName=ProxySetNtcDataX
  Data Store Read4 : DataStoreRead  DataStoreName=DiagcMgrNtcInfoXDebCntrAry
  Data Store Read5 : DataStoreRead  DataStoreName=DiagcMgrNtcInfoXDebCntrAry
  Data Store Write1 : DataStoreWrite  DataStoreName=DiagcDataX
  Data Store Write2 : DataStoreWrite  DataStoreName=DiagcMgrNtcInfoXAry
  Data Store Write3 : DataStoreWrite  DataStoreName=ProxySetNtcDataX
  Data Store Write4 : DataStoreWrite  DataStoreName=DiagcMgrNtcInfoXDebCntrAry
  Data Type Conversion : DataTypeConversion  OutDataTypeStr=uint16
  Selector : Selector  IndexMode=Zero-based  InputPortWidth=14  IndexOptions=Index vector (port)  Indices=[1 3]  OutputSizes=1
  Selector1 : Selector  IndexMode=Zero-based  InputPortWidth=512  IndexOptions=Index vector (port)  Indices=[1 3]  OutputSizes=1
  Selector2 : Selector  IndexMode=Zero-based  InputPortWidth=14  IndexOptions=Index vector (port)  Indices=[1 3]  OutputSizes=1
  SetNtcStsCore : Subsystem  Description=|  RequirementInfo={} %GIDa_4ea54909_a762_45cb_a4ed_acd11dc7d8c3
      | DOES THE STDRTN NEEDS TO BE SHOWN AS AN OUTPUT OF THE SERVER AND
      | CLIENT CALLS?
      settings: AttributesFormatString=%<Description>
  SetNtcSts_StdRtn : Outport
  wires:
  Data Store Read2/1 -> Selector1/1
  Selector1/1 -> Bus Selector3/1
  NtcNr_ArgIn/1 -> Data Type Conversion/1, SetNtcStsCore/1(NtcNr_ArgIn)
  Data Type Conversion/1 -> Selector1/2
  Bus Selector3/1 -> Assignment/3, Selector/2  "<NtcInfoIdx>"
  NtcStInfo_ArgIn/1 -> SetNtcStsCore/2(NtcStInfo_ArgIn)
  NtcSts_ArgIn/1 -> SetNtcStsCore/3(NtcSts_ArgIn)
  DebStep_ArgIn/1 -> SetNtcStsCore/4(DebStep_ArgIn)
  SetNtcStsCore/5(SetNtcSts_StdRtn) -> SetNtcSts_StdRtn/1
  SetNtcStsCore/2("DiagcDataX_ArgOut ") -> Data Store Write1/1
  SetNtcStsCore/3("ProxySetNtcDataX_ArgOut ") -> Data Store Write3/1
  Data Store Read1/1 -> SetNtcStsCore/5(DiagcDataX_ArgIn)
  Data Store Read3/1 -> SetNtcStsCore/6(ProxySetNtcDataX_ArgIn)
  Selector/1 -> SetNtcStsCore/7(DiagcMgrNtcInfoX_ArgIn)
  Data Store Read/1 -> Assignment/1, Selector/1
  Assignment/1 -> Data Store Write2/1
  SetNtcStsCore/1("NtcInfo_ArgOut ") -> Assignment/2
  Bus Selector3/2 -> Assignment1/3, Selector2/2  "<DebCntrIdx>"
  Data Store Read4/1 -> Selector2/1
  Selector2/1 -> SetNtcStsCore/8(NtcInfoDebCntrX_ArgIn)
  Assignment1/1 -> Data Store Write4/1
  SetNtcStsCore/4("NtcInfoDebCntr_ArgOut ") -> Assignment1/2
  Data Store Read5/1 -> Assignment1/1

== system ES101A_DiagcMgrProxyX/DiagcMgrProxyApplX/DiagcMgrProxyApplXInit1/CopyRight2 ==

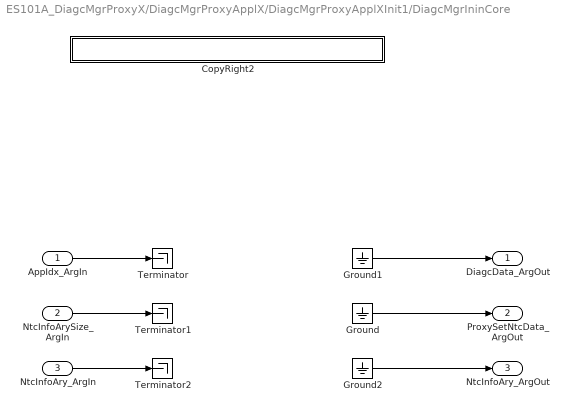
== system ES101A_DiagcMgrProxyX/DiagcMgrProxyApplX/DiagcMgrProxyApplXInit1/DiagcMgrIninCore ==
  AppIdx_ArgIn : Inport
  NtcInfoArySize_ArgIn : Inport  Port=2
  NtcInfoAry_ArgIn : Inport  Port=3
  CopyRight2 : Subsystem  Description=|  mask(Copyright Information){none=on}
      | Copyright info block.                                               
      |                                                                     
      | Place copyright information at the top of every subsystem in design.
      mask prompts: none "No parameters"
      mask help: Place copyright information at the top of every subsystem in design.
      mask Display:
      | NxtrConf = 'Nexteer Confidential';
      | 
      | sys = bdroot; %handle for the current model ("system")
      | first = get_param(sys,'Created');
      | first = first(end-3:end);  %year is last four digits
      | 
      | last = get_param(sys,'LastModifiedDate');
      | if isempty(last)
      |     last = datestr(now,'yyyy');
      | else
      |     last = last(end-3:end);
      | end
      | 
      | if strcmp(first,last)
      |     fprintf('%s -- Copyright %s Nexteer',NxtrConf,first)
      | else
      |     fprintf('%s -- %s%s- %s Nexteer',NxtrConf,char(169),first,last)
      | end
  Ground : Ground
  Ground1 : Ground
  Ground2 : Ground
  Terminator : Terminator
  Terminator1 : Terminator
  Terminator2 : Terminator
  DiagcData_ArgOut : Outport
  ProxySetNtcData_ArgOut : Outport  Port=2
  NtcInfoAry_ArgOut : Outport  Port=3
  wires:
  Ground/1 -> ProxySetNtcData_ArgOut/1
  Ground1/1 -> DiagcData_ArgOut/1
  AppIdx_ArgIn/1 -> Terminator/1
  NtcInfoArySize_ArgIn/1 -> Terminator1/1
  Ground2/1 -> NtcInfoAry_ArgOut/1
  NtcInfoAry_ArgIn/1 -> Terminator2/1

== system ES101A_DiagcMgrProxyX/DiagcMgrProxyApplX/DiagcMgrProxyApplXPer1/Clear All NTCs ==
  ClrNtcFlg : Inport
  Number of Iterations : Inport  Port=2
  Action Port : ActionPort
  CopyRight2 : Subsystem  Description=|  mask(Copyright Information){none=on}
      | Copyright info block.                                               
      |                                                                     
      | Place copyright information at the top of every subsystem in design.
      mask prompts: none "No parameters"
      mask help: Place copyright information at the top of every subsystem in design.
      mask Display:
      | NxtrConf = 'Nexteer Confidential';
      | 
      | sys = bdroot; %handle for the current model ("system")
      | first = get_param(sys,'Created');
      | first = first(end-3:end);  %year is last four digits
      | 
      | last = get_param(sys,'LastModifiedDate');
      | if isempty(last)
      |     last = datestr(now,'yyyy');
      | else
      |     last = last(end-3:end);
      | end
      | 
      | if strcmp(first,last)
      |     fprintf('%s -- Copyright %s Nexteer',NxtrConf,first)
      | else
      |     fprintf('%s -- %s%s- %s Nexteer',NxtrConf,char(169),first,last)
      | end
  Data Store Write2 : DataStoreWrite  DataStoreName=PrevClrNtcFlgX
  For Number of NTCs in NtcInfoAryX : Subsystem  Priority=1
      settings: AttributesFormatString=Priority = %<Priority>
  Initialize Proxy SetNtc and DiagcData values : Subsystem  Description=EXCLUSIVE AREA  Priority=2
      settings: AttributesFormatString=|
      | Priority = %<Priority>
      | %<Description>
  wires:
  ClrNtcFlg/1 -> Data Store Write2/1
  Number of Iterations/1 -> For Number of NTCs in NtcInfoAryX/1(Number of Iterations)

== system ES101A_DiagcMgrProxyX/DiagcMgrProxyApplX/DiagcMgrProxyApplXPer1/CopyRight2 ==

== system ES101A_DiagcMgrProxyX/DiagcMgrProxyApplX/DiagcMgrProxyApplXPer1/Update the DiagcSts ==
  Number of Iterations : Inport
  Action Port : ActionPort
  Atomic Section : Subsystem  Description=EXCLUSIVE AREA  RequirementInfo="{'linktype_rmi_doors' '0000c474 (/ESG Group/FDD Module Requirements/EA4 Specific/ES101A_DiagcMgr)' '#ES101A_290' 'true' 'REQ:  ES101A_290' '' ; 'linktype_rmi_doors' '0000c474 (/ESG Group/FDD Module Requirements/EA4 Specific/ES101A_DiagcMgr)' '#ES101A_300' 'true' 'REQ:  ES101A_300' '' } %GIDa_025ec558_e464_4c14_8c70_97d3a33a52dc"  Priority=4  TreatAsAtomicUnit=on
      settings: AttributesFormatString=|
      | Priority = %<Priority>
      | %<Description>
  CopyRight2 : Subsystem  Description=|  mask(Copyright Information){none=on}
      | Copyright info block.                                               
      |                                                                     
      | Place copyright information at the top of every subsystem in design.
      mask prompts: none "No parameters"
      mask help: Place copyright information at the top of every subsystem in design.
      mask Display:
      | NxtrConf = 'Nexteer Confidential';
      | 
      | sys = bdroot; %handle for the current model ("system")
      | first = get_param(sys,'Created');
      | first = first(end-3:end);  %year is last four digits
      | 
      | last = get_param(sys,'LastModifiedDate');
      | if isempty(last)
      |     last = datestr(now,'yyyy');
      | else
      |     last = last(end-3:end);
      | end
      | 
      | if strcmp(first,last)
      |     fprintf('%s -- Copyright %s Nexteer',NxtrConf,first)
      | else
      |     fprintf('%s -- %s%s- %s Nexteer',NxtrConf,char(169),first,last)
      | end
  For Number of NTCs : Subsystem  Priority=3  TreatAsAtomicUnit=on
      settings: AttributesFormatString=Priority = %<Priority>
  Initialize Proxy Per values : Subsystem  RequirementInfo="{'linktype_rmi_doors' '0000c474 (/ESG Group/FDD Module Requirements/EA4 Specific/ES101A_DiagcMgr)' '#ES101A_288' 'true' 'REQ:  ES101A_288' '' } %GIDa_9d8b48d1_9e1d_4477_8f3a_699616ca99a6"  Priority=2
      settings: AttributesFormatString=Priority = %<Priority>
  Initialize Proxy SetNtc values : Subsystem  Description=EXCLUSIVE AREA  RequirementInfo="{'linktype_rmi_doors' '0000c474 (/ESG Group/FDD Module Requirements/EA4 Specific/ES101A_DiagcMgr)' '#ES101A_288' 'true' 'REQ:  ES101A_288' '' } %GIDa_8de63a8f_9dfc_4051_91b0_5f7852e6f39b"  Priority=1
      settings: AttributesFormatString=|
      | Priority = %<Priority>
      | %<Description>
  wires:
  Number of Iterations/1 -> For Number of NTCs/1(Number of Iterations)

== system ES101A_DiagcMgrProxyX/DiagcMgrProxyApplX/GetDiagcDataX /CopyRight2 ==

== system ES101A_DiagcMgrProxyX/DiagcMgrProxyApplX/GetNtcActvX/CopyRight2 ==

== system ES101A_DiagcMgrProxyX/DiagcMgrProxyApplX/GetNtcActvX/GetNtcActvCore ==
  NtcNr_ArgIn : Inport
  NtcInfoAry_ArgIn : Inport  Port=2
  CopyRight2 : Subsystem  Description=|  mask(Copyright Information){none=on}
      | Copyright info block.                                               
      |                                                                     
      | Place copyright information at the top of every subsystem in design.
      mask prompts: none "No parameters"
      mask help: Place copyright information at the top of every subsystem in design.
      mask Display:
      | NxtrConf = 'Nexteer Confidential';
      | 
      | sys = bdroot; %handle for the current model ("system")
      | first = get_param(sys,'Created');
      | first = first(end-3:end);  %year is last four digits
      | 
      | last = get_param(sys,'LastModifiedDate');
      | if isempty(last)
      |     last = datestr(now,'yyyy');
      | else
      |     last = last(end-3:end);
      | end
      | 
      | if strcmp(first,last)
      |     fprintf('%s -- Copyright %s Nexteer',NxtrConf,first)
      | else
      |     fprintf('%s -- %s%s- %s Nexteer',NxtrConf,char(169),first,last)
      | end
  Ground2 : Ground
  Terminator : Terminator
  Terminator1 : Terminator
  NtcActv_ArgOut : Outport
  wires:
  NtcNr_ArgIn/1 -> Terminator/1
  NtcInfoAry_ArgIn/1 -> Terminator1/1
  Ground2/1 -> NtcActv_ArgOut/1

== system ES101A_DiagcMgrProxyX/DiagcMgrProxyApplX/GetNtcDebCntrApplX/CopyRight2 ==

== system ES101A_DiagcMgrProxyX/DiagcMgrProxyApplX/GetNtcInfoAppIX/CopyRight2 ==

== system ES101A_DiagcMgrProxyX/DiagcMgrProxyApplX/GetNtcQlfrStsX/CopyRight2 ==

== system ES101A_DiagcMgrProxyX/DiagcMgrProxyApplX/GetNtcQlfrStsX/GetNtcQlfrStsCore ==
  NtcNr_ArgIn : Inport
  NtcInfoAry_ArgIn : Inport  Port=2
  CopyRight2 : Subsystem  Description=|  mask(Copyright Information){none=on}
      | Copyright info block.                                               
      |                                                                     
      | Place copyright information at the top of every subsystem in design.
      mask prompts: none "No parameters"
      mask help: Place copyright information at the top of every subsystem in design.
      mask Display:
      | NxtrConf = 'Nexteer Confidential';
      | 
      | sys = bdroot; %handle for the current model ("system")
      | first = get_param(sys,'Created');
      | first = first(end-3:end);  %year is last four digits
      | 
      | last = get_param(sys,'LastModifiedDate');
      | if isempty(last)
      |     last = datestr(now,'yyyy');
      | else
      |     last = last(end-3:end);
      | end
      | 
      | if strcmp(first,last)
      |     fprintf('%s -- Copyright %s Nexteer',NxtrConf,first)
      | else
      |     fprintf('%s -- %s%s- %s Nexteer',NxtrConf,char(169),first,last)
      | end
  Ground2 : Ground
  Terminator : Terminator
  Terminator1 : Terminator
  NtcQlfr_ArgOut : Outport
  wires:
  Ground2/1 -> NtcQlfr_ArgOut/1
  NtcInfoAry_ArgIn/1 -> Terminator1/1
  NtcNr_ArgIn/1 -> Terminator/1

== system ES101A_DiagcMgrProxyX/DiagcMgrProxyApplX/GetNtcStsX/CopyRight2 ==

== system ES101A_DiagcMgrProxyX/DiagcMgrProxyApplX/GetNtcStsX/GetNtcStsCore ==
  NtcNr_ArgIn : Inport
  NtcInfoAry_ArgIn : Inport  Port=2
  CopyRight2 : Subsystem  Description=|  mask(Copyright Information){none=on}
      | Copyright info block.                                               
      |                                                                     
      | Place copyright information at the top of every subsystem in design.
      mask prompts: none "No parameters"
      mask help: Place copyright information at the top of every subsystem in design.
      mask Display:
      | NxtrConf = 'Nexteer Confidential';
      | 
      | sys = bdroot; %handle for the current model ("system")
      | first = get_param(sys,'Created');
      | first = first(end-3:end);  %year is last four digits
      | 
      | last = get_param(sys,'LastModifiedDate');
      | if isempty(last)
      |     last = datestr(now,'yyyy');
      | else
      |     last = last(end-3:end);
      | end
      | 
      | if strcmp(first,last)
      |     fprintf('%s -- Copyright %s Nexteer',NxtrConf,first)
      | else
      |     fprintf('%s -- %s%s- %s Nexteer',NxtrConf,char(169),first,last)
      | end
  Ground2 : Ground
  Terminator : Terminator
  Terminator1 : Terminator
  NtcInfoSts_ArgOut : Outport
  wires:
  NtcNr_ArgIn/1 -> Terminator/1
  NtcInfoAry_ArgIn/1 -> Terminator1/1
  Ground2/1 -> NtcInfoSts_ArgOut/1

== system ES101A_DiagcMgrProxyX/DiagcMgrProxyApplX/SetNtcStsX/CopyRight2 ==
